simulink model "lab5"  (R2018b)
settings: Solver=VariableStepAuto  StartTime=0.0  StopTime=10.0  RelTol=1e-3
values from neighbouring files (symbols this model uses):
  b = fir2(8,f,m)    [Untitled3.m]
libraries: dspsrcs4 x2, dspsnks4 x1, dspvision x1, dspfdesign x1
settings Model: Creator=Student  LastModifiedBy=Student

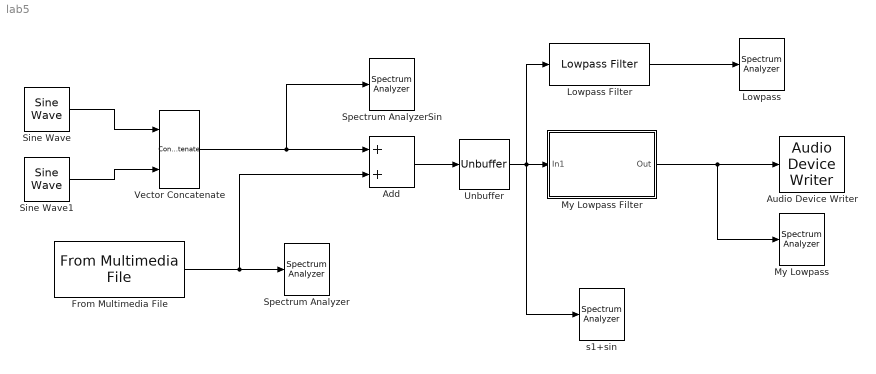
== system lab5 ==
  Add : Sum
  Audio Device Writer : dspsnks4/Audio Device Writer  Driver=DirectSound  Device=Default  InheritSampleRate=on  SampleRate=44100  BitDepth=16-bit integer  BufferSize=4096  NumBuffers=10  DefaultOutputChannelMapping=on  OutputChannelMapping=1:2  OutputNumUnderrunSamples=off  DriverIdx=1  DeviceWarnFlag=''
  From Multimedia File : dspvision/From Multimedia File  inputFilename=C:\Users\student\Documents\MATLAB\S1.mp3  loop=on  numPlays=inf  outputStreams=Audio only  videoDataType=single  audioDataType=double  inheritSampleTime=on  userDefinedSampleTime=1/30  noAudioOutput=off  isIntensityVideo=off  fourcc=RGB  colorVideoFormat=Separate color signals  outputEOF=off  dataOrg=Column-major  audioFrameSize=1024  computeAudioFrameSize=off  outSamplingMode=Sample based
      settings: SourceProductBaseCode=VP
  Lowpass : SpectrumAnalyzer
  Lowpass Filter : dspfdesign/Lowpass Filter  FilterType=FIR  DesignForMinimumOrder=on  FilterOrder=50  PassbandFrequency=8e3  StopbandFrequency=12e3  PassbandRipple=0.1  StopbandAttenuation=80  InheritSampleRate=off  SampleRate=44100  SimulateUsing=Interpreted execution  roundingMode=Floor  coeffsDataTypeStr=fixdt(1,16)
  My Lowpass : SpectrumAnalyzer
  "My Lowpass Filter " : Subsystem
  Sine Wave : dspsrcs4/Sine Wave  Amplitude=1  Frequency=17000  Phase=0  SampleMode=Discrete  OutComplex=Real  CompMethod=Trigonometric fcn  TableSize=Speed  SampleTime=1/44100  SamplesPerFrame=1024  ResetState=Restart at time zero  OutputFrames=off  dataType=double  wordLen=16  udDataType=sfix(16)  fracBitsMode=Best precision  numFracBits=15  OutDataTypeStr=double  LastOutDataTypeStr=double
  Sine Wave1 : dspsrcs4/Sine Wave  Amplitude=1  Frequency=17000  Phase=0  SampleMode=Discrete  OutComplex=Real  CompMethod=Trigonometric fcn  TableSize=Speed  SampleTime=1/44100  SamplesPerFrame=1024  ResetState=Restart at time zero  OutputFrames=off  dataType=double  wordLen=16  udDataType=sfix(16)  fracBitsMode=Best precision  numFracBits=15  OutDataTypeStr=double  LastOutDataTypeStr=double
  Spectrum Analyzer : SpectrumAnalyzer
  Spectrum AnalyzerSin : SpectrumAnalyzer
  Unbuffer : Unbuffer
  Vector Concatenate : Concatenate  Mode=Multidimensional array  ConcatenateDimension=2
  s1+sin : SpectrumAnalyzer
  wires:
  Add/1 -> Unbuffer/1
  Unbuffer/1 -> Lowpass Filter/1, s1+sin/1, "My Lowpass Filter "/1(In1)
  From Multimedia File/1 -> Spectrum Analyzer/1, Add/2
  Sine Wave/1 -> Vector Concatenate/1
  Sine Wave1/1 -> Vector Concatenate/2
  Vector Concatenate/1 -> Spectrum AnalyzerSin/1, Add/1
  "My Lowpass Filter "/1(Out) -> My Lowpass/1, Audio Device Writer/1
  Lowpass Filter/1 -> Lowpass/1

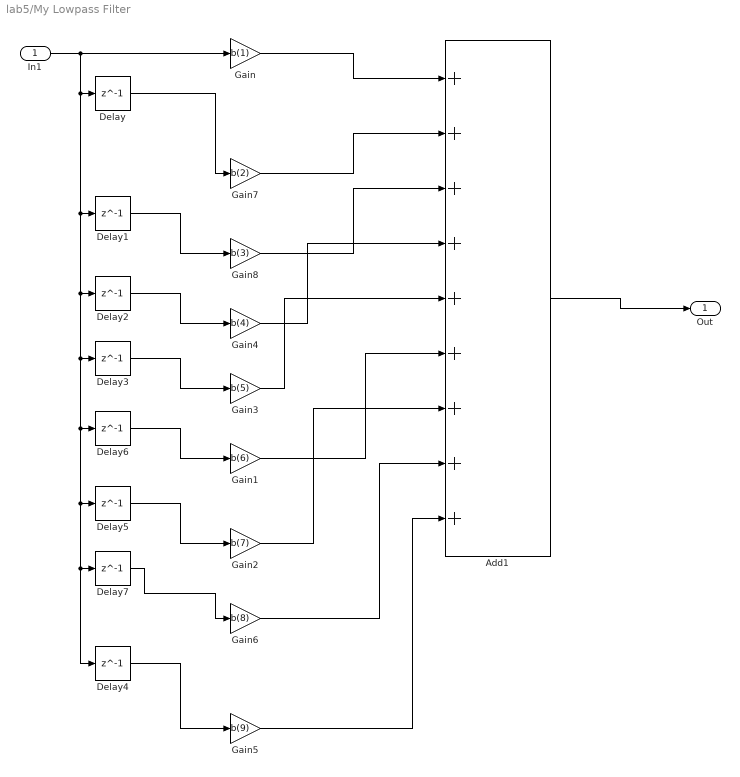
== system lab5/My Lowpass Filter  ==
  In1 : Inport
  Add1 : Sum  Inputs=+++++++++
  Delay{,1..7} (8 alike) : Delay  DelayLength=1  InitialCondition=0
  Gain : Gain  Gain=b(1)
  Gain1 : Gain  Gain=b(6)
  Gain2 : Gain  Gain=b(7)
  Gain3 : Gain  Gain=b(5)
  Gain4 : Gain  Gain=b(4)
  Gain5 : Gain  Gain=b(9)
  Gain6 : Gain  Gain=b(8)
  Gain7 : Gain  Gain=b(2)
  Gain8 : Gain  Gain=b(3)
  Out : Outport
  wires:
  Gain2/1 -> Add1/7
  Delay5/1 -> Gain2/1
  Add1/1 -> Out/1
  Gain8/1 -> Add1/3
  In1/1 -> Delay4/1, Delay7/1, Delay5/1, Delay6/1, Delay3/1, Delay2/1, Delay1/1, Delay/1, Gain/1
  Gain1/1 -> Add1/6
  ? -> ?
  Gain7/1 -> Add1/2
  Delay3/1 -> Gain3/1
  Delay/1 -> Gain7/1
  Gain/1 -> Add1/1
  Gain6/1 -> Add1/8
  Gain5/1 -> Add1/9
  Gain4/1 -> Add1/4
  Gain3/1 -> Add1/5
  Delay6/1 -> Gain1/1
  Delay7/1 -> Gain6/1
  Delay2/1 -> Gain4/1
  Delay1/1 -> Gain8/1
  Delay4/1 -> Gain5/1
